simulink model "lab7_1"  (R2018b)
settings: Solver=VariableStepAuto  StartTime=0.0  StopTime=10.0  RelTol=1e-3
libraries: hdlsllib x86
(part 2 of 2)

== system lab7_1/Subsystem1/Full Adder2/Half Adder 1 ==
  note: Subsystem
  X : Inport
  Y : Inport  Port=2
  Logical Operator : Logic  IconShape=distinctive  AllPortsSameDT=off  OutDataTypeStr=boolean
  Logical Operator1 : Logic  Operator=XOR  IconShape=distinctive  AllPortsSameDT=off  OutDataTypeStr=boolean
  S : Outport
  C : Outport  Port=2
  wires:
  X/1 -> Logical Operator/1, Logical Operator1/1
  Y/1 -> Logical Operator1/2, Logical Operator/2
  Logical Operator/1 -> C/1
  Logical Operator1/1 -> S/1

== system lab7_1/Subsystem1/Full Adder3/Half Adder ==
  note: Subsystem
  X : Inport
  Y : Inport  Port=2
  Logical Operator : Logic  IconShape=distinctive  AllPortsSameDT=off  OutDataTypeStr=boolean
  Logical Operator1 : Logic  Operator=XOR  IconShape=distinctive  AllPortsSameDT=off  OutDataTypeStr=boolean
  S : Outport
  C : Outport  Port=2
  wires:
  X/1 -> Logical Operator/1, Logical Operator1/1
  Y/1 -> Logical Operator1/2, Logical Operator/2
  Logical Operator/1 -> C/1
  Logical Operator1/1 -> S/1

== system lab7_1/Subsystem1/Full Adder3/Half Adder 1 ==
  note: Subsystem
  X : Inport
  Y : Inport  Port=2
  Logical Operator : Logic  IconShape=distinctive  AllPortsSameDT=off  OutDataTypeStr=boolean
  Logical Operator1 : Logic  Operator=XOR  IconShape=distinctive  AllPortsSameDT=off  OutDataTypeStr=boolean
  S : Outport
  C : Outport  Port=2
  wires:
  X/1 -> Logical Operator/1, Logical Operator1/1
  Y/1 -> Logical Operator1/2, Logical Operator/2
  Logical Operator/1 -> C/1
  Logical Operator1/1 -> S/1

== system lab7_1/Subsystem1/Full Adder4/Half Adder ==
  note: Subsystem
  X : Inport
  Y : Inport  Port=2
  Logical Operator : Logic  IconShape=distinctive  AllPortsSameDT=off  OutDataTypeStr=boolean
  Logical Operator1 : Logic  Operator=XOR  IconShape=distinctive  AllPortsSameDT=off  OutDataTypeStr=boolean
  S : Outport
  C : Outport  Port=2
  wires:
  X/1 -> Logical Operator/1, Logical Operator1/1
  Y/1 -> Logical Operator1/2, Logical Operator/2
  Logical Operator/1 -> C/1
  Logical Operator1/1 -> S/1

== system lab7_1/Subsystem1/Full Adder4/Half Adder 1 ==
  note: Subsystem
  X : Inport
  Y : Inport  Port=2
  Logical Operator : Logic  IconShape=distinctive  AllPortsSameDT=off  OutDataTypeStr=boolean
  Logical Operator1 : Logic  Operator=XOR  IconShape=distinctive  AllPortsSameDT=off  OutDataTypeStr=boolean
  S : Outport
  C : Outport  Port=2
  wires:
  X/1 -> Logical Operator/1, Logical Operator1/1
  Y/1 -> Logical Operator1/2, Logical Operator/2
  Logical Operator/1 -> C/1
  Logical Operator1/1 -> S/1

== system lab7_1/Subsystem1/Full Adder5/Half Adder ==
  note: Subsystem
  X : Inport
  Y : Inport  Port=2
  Logical Operator : Logic  IconShape=distinctive  AllPortsSameDT=off  OutDataTypeStr=boolean
  Logical Operator1 : Logic  Operator=XOR  IconShape=distinctive  AllPortsSameDT=off  OutDataTypeStr=boolean
  S : Outport
  C : Outport  Port=2
  wires:
  X/1 -> Logical Operator/1, Logical Operator1/1
  Y/1 -> Logical Operator1/2, Logical Operator/2
  Logical Operator/1 -> C/1
  Logical Operator1/1 -> S/1

== system lab7_1/Subsystem1/Full Adder5/Half Adder 1 ==
  note: Subsystem
  X : Inport
  Y : Inport  Port=2
  Logical Operator : Logic  IconShape=distinctive  AllPortsSameDT=off  OutDataTypeStr=boolean
  Logical Operator1 : Logic  Operator=XOR  IconShape=distinctive  AllPortsSameDT=off  OutDataTypeStr=boolean
  S : Outport
  C : Outport  Port=2
  wires:
  X/1 -> Logical Operator/1, Logical Operator1/1
  Y/1 -> Logical Operator1/2, Logical Operator/2
  Logical Operator/1 -> C/1
  Logical Operator1/1 -> S/1

== system lab7_1/Subsystem1/Full Adder6/Half Adder ==
  note: Subsystem
  X : Inport
  Y : Inport  Port=2
  Logical Operator : Logic  IconShape=distinctive  AllPortsSameDT=off  OutDataTypeStr=boolean
  Logical Operator1 : Logic  Operator=XOR  IconShape=distinctive  AllPortsSameDT=off  OutDataTypeStr=boolean
  S : Outport
  C : Outport  Port=2
  wires:
  X/1 -> Logical Operator/1, Logical Operator1/1
  Y/1 -> Logical Operator1/2, Logical Operator/2
  Logical Operator/1 -> C/1
  Logical Operator1/1 -> S/1

== system lab7_1/Subsystem1/Full Adder6/Half Adder 1 ==
  note: Subsystem
  X : Inport
  Y : Inport  Port=2
  Logical Operator : Logic  IconShape=distinctive  AllPortsSameDT=off  OutDataTypeStr=boolean
  Logical Operator1 : Logic  Operator=XOR  IconShape=distinctive  AllPortsSameDT=off  OutDataTypeStr=boolean
  S : Outport
  C : Outport  Port=2
  wires:
  X/1 -> Logical Operator/1, Logical Operator1/1
  Y/1 -> Logical Operator1/2, Logical Operator/2
  Logical Operator/1 -> C/1
  Logical Operator1/1 -> S/1

== system lab7_1/Subsystem1/Full Adder7/Half Adder ==
  note: Subsystem
  X : Inport
  Y : Inport  Port=2
  Logical Operator : Logic  IconShape=distinctive  AllPortsSameDT=off  OutDataTypeStr=boolean
  Logical Operator1 : Logic  Operator=XOR  IconShape=distinctive  AllPortsSameDT=off  OutDataTypeStr=boolean
  S : Outport
  C : Outport  Port=2
  wires:
  X/1 -> Logical Operator/1, Logical Operator1/1
  Y/1 -> Logical Operator1/2, Logical Operator/2
  Logical Operator/1 -> C/1
  Logical Operator1/1 -> S/1

== system lab7_1/Subsystem1/Full Adder7/Half Adder 1 ==
  note: Subsystem
  X : Inport
  Y : Inport  Port=2
  Logical Operator : Logic  IconShape=distinctive  AllPortsSameDT=off  OutDataTypeStr=boolean
  Logical Operator1 : Logic  Operator=XOR  IconShape=distinctive  AllPortsSameDT=off  OutDataTypeStr=boolean
  S : Outport
  C : Outport  Port=2
  wires:
  X/1 -> Logical Operator/1, Logical Operator1/1
  Y/1 -> Logical Operator1/2, Logical Operator/2
  Logical Operator/1 -> C/1
  Logical Operator1/1 -> S/1

== system lab7_1/Subsystem2/Full Adder/Half Adder ==
  note: Subsystem
  X : Inport
  Y : Inport  Port=2
  Logical Operator : Logic  IconShape=distinctive  AllPortsSameDT=off  OutDataTypeStr=boolean
  Logical Operator1 : Logic  Operator=XOR  IconShape=distinctive  AllPortsSameDT=off  OutDataTypeStr=boolean
  S : Outport
  C : Outport  Port=2
  wires:
  X/1 -> Logical Operator/1, Logical Operator1/1
  Y/1 -> Logical Operator1/2, Logical Operator/2
  Logical Operator/1 -> C/1
  Logical Operator1/1 -> S/1

== system lab7_1/Subsystem2/Full Adder/Half Adder 1 ==
  note: Subsystem
  X : Inport
  Y : Inport  Port=2
  Logical Operator : Logic  IconShape=distinctive  AllPortsSameDT=off  OutDataTypeStr=boolean
  Logical Operator1 : Logic  Operator=XOR  IconShape=distinctive  AllPortsSameDT=off  OutDataTypeStr=boolean
  S : Outport
  C : Outport  Port=2
  wires:
  X/1 -> Logical Operator/1, Logical Operator1/1
  Y/1 -> Logical Operator1/2, Logical Operator/2
  Logical Operator/1 -> C/1
  Logical Operator1/1 -> S/1

== system lab7_1/Subsystem2/Full Adder1/Half Adder ==
  note: Subsystem
  X : Inport
  Y : Inport  Port=2
  Logical Operator : Logic  IconShape=distinctive  AllPortsSameDT=off  OutDataTypeStr=boolean
  Logical Operator1 : Logic  Operator=XOR  IconShape=distinctive  AllPortsSameDT=off  OutDataTypeStr=boolean
  S : Outport
  C : Outport  Port=2
  wires:
  X/1 -> Logical Operator/1, Logical Operator1/1
  Y/1 -> Logical Operator1/2, Logical Operator/2
  Logical Operator/1 -> C/1
  Logical Operator1/1 -> S/1

== system lab7_1/Subsystem2/Full Adder1/Half Adder 1 ==
  note: Subsystem
  X : Inport
  Y : Inport  Port=2
  Logical Operator : Logic  IconShape=distinctive  AllPortsSameDT=off  OutDataTypeStr=boolean
  Logical Operator1 : Logic  Operator=XOR  IconShape=distinctive  AllPortsSameDT=off  OutDataTypeStr=boolean
  S : Outport
  C : Outport  Port=2
  wires:
  X/1 -> Logical Operator/1, Logical Operator1/1
  Y/1 -> Logical Operator1/2, Logical Operator/2
  Logical Operator/1 -> C/1
  Logical Operator1/1 -> S/1

== system lab7_1/Subsystem2/Full Adder2/Half Adder ==
  note: Subsystem
  X : Inport
  Y : Inport  Port=2
  Logical Operator : Logic  IconShape=distinctive  AllPortsSameDT=off  OutDataTypeStr=boolean
  Logical Operator1 : Logic  Operator=XOR  IconShape=distinctive  AllPortsSameDT=off  OutDataTypeStr=boolean
  S : Outport
  C : Outport  Port=2
  wires:
  X/1 -> Logical Operator/1, Logical Operator1/1
  Y/1 -> Logical Operator1/2, Logical Operator/2
  Logical Operator/1 -> C/1
  Logical Operator1/1 -> S/1

== system lab7_1/Subsystem2/Full Adder2/Half Adder 1 ==
  note: Subsystem
  X : Inport
  Y : Inport  Port=2
  Logical Operator : Logic  IconShape=distinctive  AllPortsSameDT=off  OutDataTypeStr=boolean
  Logical Operator1 : Logic  Operator=XOR  IconShape=distinctive  AllPortsSameDT=off  OutDataTypeStr=boolean
  S : Outport
  C : Outport  Port=2
  wires:
  X/1 -> Logical Operator/1, Logical Operator1/1
  Y/1 -> Logical Operator1/2, Logical Operator/2
  Logical Operator/1 -> C/1
  Logical Operator1/1 -> S/1

== system lab7_1/Subsystem2/Full Adder3/Half Adder ==
  note: Subsystem
  X : Inport
  Y : Inport  Port=2
  Logical Operator : Logic  IconShape=distinctive  AllPortsSameDT=off  OutDataTypeStr=boolean
  Logical Operator1 : Logic  Operator=XOR  IconShape=distinctive  AllPortsSameDT=off  OutDataTypeStr=boolean
  S : Outport
  C : Outport  Port=2
  wires:
  X/1 -> Logical Operator/1, Logical Operator1/1
  Y/1 -> Logical Operator1/2, Logical Operator/2
  Logical Operator/1 -> C/1
  Logical Operator1/1 -> S/1

== system lab7_1/Subsystem2/Full Adder3/Half Adder 1 ==
  note: Subsystem
  X : Inport
  Y : Inport  Port=2
  Logical Operator : Logic  IconShape=distinctive  AllPortsSameDT=off  OutDataTypeStr=boolean
  Logical Operator1 : Logic  Operator=XOR  IconShape=distinctive  AllPortsSameDT=off  OutDataTypeStr=boolean
  S : Outport
  C : Outport  Port=2
  wires:
  X/1 -> Logical Operator/1, Logical Operator1/1
  Y/1 -> Logical Operator1/2, Logical Operator/2
  Logical Operator/1 -> C/1
  Logical Operator1/1 -> S/1

== system lab7_1/Subsystem2/Full Adder4/Half Adder ==
  note: Subsystem
  X : Inport
  Y : Inport  Port=2
  Logical Operator : Logic  IconShape=distinctive  AllPortsSameDT=off  OutDataTypeStr=boolean
  Logical Operator1 : Logic  Operator=XOR  IconShape=distinctive  AllPortsSameDT=off  OutDataTypeStr=boolean
  S : Outport
  C : Outport  Port=2
  wires:
  X/1 -> Logical Operator/1, Logical Operator1/1
  Y/1 -> Logical Operator1/2, Logical Operator/2
  Logical Operator/1 -> C/1
  Logical Operator1/1 -> S/1

== system lab7_1/Subsystem2/Full Adder4/Half Adder 1 ==
  note: Subsystem
  X : Inport
  Y : Inport  Port=2
  Logical Operator : Logic  IconShape=distinctive  AllPortsSameDT=off  OutDataTypeStr=boolean
  Logical Operator1 : Logic  Operator=XOR  IconShape=distinctive  AllPortsSameDT=off  OutDataTypeStr=boolean
  S : Outport
  C : Outport  Port=2
  wires:
  X/1 -> Logical Operator/1, Logical Operator1/1
  Y/1 -> Logical Operator1/2, Logical Operator/2
  Logical Operator/1 -> C/1
  Logical Operator1/1 -> S/1

== system lab7_1/Subsystem2/Full Adder5/Half Adder ==
  note: Subsystem
  X : Inport
  Y : Inport  Port=2
  Logical Operator : Logic  IconShape=distinctive  AllPortsSameDT=off  OutDataTypeStr=boolean
  Logical Operator1 : Logic  Operator=XOR  IconShape=distinctive  AllPortsSameDT=off  OutDataTypeStr=boolean
  S : Outport
  C : Outport  Port=2
  wires:
  X/1 -> Logical Operator/1, Logical Operator1/1
  Y/1 -> Logical Operator1/2, Logical Operator/2
  Logical Operator/1 -> C/1
  Logical Operator1/1 -> S/1

== system lab7_1/Subsystem2/Full Adder5/Half Adder 1 ==
  note: Subsystem
  X : Inport
  Y : Inport  Port=2
  Logical Operator : Logic  IconShape=distinctive  AllPortsSameDT=off  OutDataTypeStr=boolean
  Logical Operator1 : Logic  Operator=XOR  IconShape=distinctive  AllPortsSameDT=off  OutDataTypeStr=boolean
  S : Outport
  C : Outport  Port=2
  wires:
  X/1 -> Logical Operator/1, Logical Operator1/1
  Y/1 -> Logical Operator1/2, Logical Operator/2
  Logical Operator/1 -> C/1
  Logical Operator1/1 -> S/1

== system lab7_1/Subsystem2/Full Adder6/Half Adder ==
  note: Subsystem
  X : Inport
  Y : Inport  Port=2
  Logical Operator : Logic  IconShape=distinctive  AllPortsSameDT=off  OutDataTypeStr=boolean
  Logical Operator1 : Logic  Operator=XOR  IconShape=distinctive  AllPortsSameDT=off  OutDataTypeStr=boolean
  S : Outport
  C : Outport  Port=2
  wires:
  X/1 -> Logical Operator/1, Logical Operator1/1
  Y/1 -> Logical Operator1/2, Logical Operator/2
  Logical Operator/1 -> C/1
  Logical Operator1/1 -> S/1

== system lab7_1/Subsystem2/Full Adder6/Half Adder 1 ==
  note: Subsystem
  X : Inport
  Y : Inport  Port=2
  Logical Operator : Logic  IconShape=distinctive  AllPortsSameDT=off  OutDataTypeStr=boolean
  Logical Operator1 : Logic  Operator=XOR  IconShape=distinctive  AllPortsSameDT=off  OutDataTypeStr=boolean
  S : Outport
  C : Outport  Port=2
  wires:
  X/1 -> Logical Operator/1, Logical Operator1/1
  Y/1 -> Logical Operator1/2, Logical Operator/2
  Logical Operator/1 -> C/1
  Logical Operator1/1 -> S/1

== system lab7_1/Subsystem2/Full Adder7/Half Adder ==
  note: Subsystem
  X : Inport
  Y : Inport  Port=2
  Logical Operator : Logic  IconShape=distinctive  AllPortsSameDT=off  OutDataTypeStr=boolean
  Logical Operator1 : Logic  Operator=XOR  IconShape=distinctive  AllPortsSameDT=off  OutDataTypeStr=boolean
  S : Outport
  C : Outport  Port=2
  wires:
  X/1 -> Logical Operator/1, Logical Operator1/1
  Y/1 -> Logical Operator1/2, Logical Operator/2
  Logical Operator/1 -> C/1
  Logical Operator1/1 -> S/1

== system lab7_1/Subsystem2/Full Adder7/Half Adder 1 ==
  note: Subsystem
  X : Inport
  Y : Inport  Port=2
  Logical Operator : Logic  IconShape=distinctive  AllPortsSameDT=off  OutDataTypeStr=boolean
  Logical Operator1 : Logic  Operator=XOR  IconShape=distinctive  AllPortsSameDT=off  OutDataTypeStr=boolean
  S : Outport
  C : Outport  Port=2
  wires:
  X/1 -> Logical Operator/1, Logical Operator1/1
  Y/1 -> Logical Operator1/2, Logical Operator/2
  Logical Operator/1 -> C/1
  Logical Operator1/1 -> S/1

== system lab7_1/Subsystem3/Full Adder/Half Adder ==
  note: Subsystem
  X : Inport
  Y : Inport  Port=2
  Logical Operator : Logic  IconShape=distinctive  AllPortsSameDT=off  OutDataTypeStr=boolean
  Logical Operator1 : Logic  Operator=XOR  IconShape=distinctive  AllPortsSameDT=off  OutDataTypeStr=boolean
  S : Outport
  C : Outport  Port=2
  wires:
  X/1 -> Logical Operator/1, Logical Operator1/1
  Y/1 -> Logical Operator1/2, Logical Operator/2
  Logical Operator/1 -> C/1
  Logical Operator1/1 -> S/1

== system lab7_1/Subsystem3/Full Adder/Half Adder 1 ==
  note: Subsystem
  X : Inport
  Y : Inport  Port=2
  Logical Operator : Logic  IconShape=distinctive  AllPortsSameDT=off  OutDataTypeStr=boolean
  Logical Operator1 : Logic  Operator=XOR  IconShape=distinctive  AllPortsSameDT=off  OutDataTypeStr=boolean
  S : Outport
  C : Outport  Port=2
  wires:
  X/1 -> Logical Operator/1, Logical Operator1/1
  Y/1 -> Logical Operator1/2, Logical Operator/2
  Logical Operator/1 -> C/1
  Logical Operator1/1 -> S/1

== system lab7_1/Subsystem3/Full Adder1/Half Adder ==
  note: Subsystem
  X : Inport
  Y : Inport  Port=2
  Logical Operator : Logic  IconShape=distinctive  AllPortsSameDT=off  OutDataTypeStr=boolean
  Logical Operator1 : Logic  Operator=XOR  IconShape=distinctive  AllPortsSameDT=off  OutDataTypeStr=boolean
  S : Outport
  C : Outport  Port=2
  wires:
  X/1 -> Logical Operator/1, Logical Operator1/1
  Y/1 -> Logical Operator1/2, Logical Operator/2
  Logical Operator/1 -> C/1
  Logical Operator1/1 -> S/1

== system lab7_1/Subsystem3/Full Adder1/Half Adder 1 ==
  note: Subsystem
  X : Inport
  Y : Inport  Port=2
  Logical Operator : Logic  IconShape=distinctive  AllPortsSameDT=off  OutDataTypeStr=boolean
  Logical Operator1 : Logic  Operator=XOR  IconShape=distinctive  AllPortsSameDT=off  OutDataTypeStr=boolean
  S : Outport
  C : Outport  Port=2
  wires:
  X/1 -> Logical Operator/1, Logical Operator1/1
  Y/1 -> Logical Operator1/2, Logical Operator/2
  Logical Operator/1 -> C/1
  Logical Operator1/1 -> S/1

== system lab7_1/Subsystem3/Full Adder2/Half Adder ==
  note: Subsystem
  X : Inport
  Y : Inport  Port=2
  Logical Operator : Logic  IconShape=distinctive  AllPortsSameDT=off  OutDataTypeStr=boolean
  Logical Operator1 : Logic  Operator=XOR  IconShape=distinctive  AllPortsSameDT=off  OutDataTypeStr=boolean
  S : Outport
  C : Outport  Port=2
  wires:
  X/1 -> Logical Operator/1, Logical Operator1/1
  Y/1 -> Logical Operator1/2, Logical Operator/2
  Logical Operator/1 -> C/1
  Logical Operator1/1 -> S/1

== system lab7_1/Subsystem3/Full Adder2/Half Adder 1 ==
  note: Subsystem
  X : Inport
  Y : Inport  Port=2
  Logical Operator : Logic  IconShape=distinctive  AllPortsSameDT=off  OutDataTypeStr=boolean
  Logical Operator1 : Logic  Operator=XOR  IconShape=distinctive  AllPortsSameDT=off  OutDataTypeStr=boolean
  S : Outport
  C : Outport  Port=2
  wires:
  X/1 -> Logical Operator/1, Logical Operator1/1
  Y/1 -> Logical Operator1/2, Logical Operator/2
  Logical Operator/1 -> C/1
  Logical Operator1/1 -> S/1

== system lab7_1/Subsystem3/Full Adder3/Half Adder ==
  note: Subsystem
  X : Inport
  Y : Inport  Port=2
  Logical Operator : Logic  IconShape=distinctive  AllPortsSameDT=off  OutDataTypeStr=boolean
  Logical Operator1 : Logic  Operator=XOR  IconShape=distinctive  AllPortsSameDT=off  OutDataTypeStr=boolean
  S : Outport
  C : Outport  Port=2
  wires:
  X/1 -> Logical Operator/1, Logical Operator1/1
  Y/1 -> Logical Operator1/2, Logical Operator/2
  Logical Operator/1 -> C/1
  Logical Operator1/1 -> S/1

== system lab7_1/Subsystem3/Full Adder3/Half Adder 1 ==
  note: Subsystem
  X : Inport
  Y : Inport  Port=2
  Logical Operator : Logic  IconShape=distinctive  AllPortsSameDT=off  OutDataTypeStr=boolean
  Logical Operator1 : Logic  Operator=XOR  IconShape=distinctive  AllPortsSameDT=off  OutDataTypeStr=boolean
  S : Outport
  C : Outport  Port=2
  wires:
  X/1 -> Logical Operator/1, Logical Operator1/1
  Y/1 -> Logical Operator1/2, Logical Operator/2
  Logical Operator/1 -> C/1
  Logical Operator1/1 -> S/1

== system lab7_1/Subsystem3/Full Adder4/Half Adder ==
  note: Subsystem
  X : Inport
  Y : Inport  Port=2
  Logical Operator : Logic  IconShape=distinctive  AllPortsSameDT=off  OutDataTypeStr=boolean
  Logical Operator1 : Logic  Operator=XOR  IconShape=distinctive  AllPortsSameDT=off  OutDataTypeStr=boolean
  S : Outport
  C : Outport  Port=2
  wires:
  X/1 -> Logical Operator/1, Logical Operator1/1
  Y/1 -> Logical Operator1/2, Logical Operator/2
  Logical Operator/1 -> C/1
  Logical Operator1/1 -> S/1

== system lab7_1/Subsystem3/Full Adder4/Half Adder 1 ==
  note: Subsystem
  X : Inport
  Y : Inport  Port=2
  Logical Operator : Logic  IconShape=distinctive  AllPortsSameDT=off  OutDataTypeStr=boolean
  Logical Operator1 : Logic  Operator=XOR  IconShape=distinctive  AllPortsSameDT=off  OutDataTypeStr=boolean
  S : Outport
  C : Outport  Port=2
  wires:
  X/1 -> Logical Operator/1, Logical Operator1/1
  Y/1 -> Logical Operator1/2, Logical Operator/2
  Logical Operator/1 -> C/1
  Logical Operator1/1 -> S/1

== system lab7_1/Subsystem3/Full Adder5/Half Adder ==
  note: Subsystem
  X : Inport
  Y : Inport  Port=2
  Logical Operator : Logic  IconShape=distinctive  AllPortsSameDT=off  OutDataTypeStr=boolean
  Logical Operator1 : Logic  Operator=XOR  IconShape=distinctive  AllPortsSameDT=off  OutDataTypeStr=boolean
  S : Outport
  C : Outport  Port=2
  wires:
  X/1 -> Logical Operator/1, Logical Operator1/1
  Y/1 -> Logical Operator1/2, Logical Operator/2
  Logical Operator/1 -> C/1
  Logical Operator1/1 -> S/1

== system lab7_1/Subsystem3/Full Adder5/Half Adder 1 ==
  note: Subsystem
  X : Inport
  Y : Inport  Port=2
  Logical Operator : Logic  IconShape=distinctive  AllPortsSameDT=off  OutDataTypeStr=boolean
  Logical Operator1 : Logic  Operator=XOR  IconShape=distinctive  AllPortsSameDT=off  OutDataTypeStr=boolean
  S : Outport
  C : Outport  Port=2
  wires:
  X/1 -> Logical Operator/1, Logical Operator1/1
  Y/1 -> Logical Operator1/2, Logical Operator/2
  Logical Operator/1 -> C/1
  Logical Operator1/1 -> S/1

== system lab7_1/Subsystem3/Full Adder6/Half Adder ==
  note: Subsystem
  X : Inport
  Y : Inport  Port=2
  Logical Operator : Logic  IconShape=distinctive  AllPortsSameDT=off  OutDataTypeStr=boolean
  Logical Operator1 : Logic  Operator=XOR  IconShape=distinctive  AllPortsSameDT=off  OutDataTypeStr=boolean
  S : Outport
  C : Outport  Port=2
  wires:
  X/1 -> Logical Operator/1, Logical Operator1/1
  Y/1 -> Logical Operator1/2, Logical Operator/2
  Logical Operator/1 -> C/1
  Logical Operator1/1 -> S/1

== system lab7_1/Subsystem3/Full Adder6/Half Adder 1 ==
  note: Subsystem
  X : Inport
  Y : Inport  Port=2
  Logical Operator : Logic  IconShape=distinctive  AllPortsSameDT=off  OutDataTypeStr=boolean
  Logical Operator1 : Logic  Operator=XOR  IconShape=distinctive  AllPortsSameDT=off  OutDataTypeStr=boolean
  S : Outport
  C : Outport  Port=2
  wires:
  X/1 -> Logical Operator/1, Logical Operator1/1
  Y/1 -> Logical Operator1/2, Logical Operator/2
  Logical Operator/1 -> C/1
  Logical Operator1/1 -> S/1

== system lab7_1/Subsystem3/Full Adder7/Half Adder ==
  note: Subsystem
  X : Inport
  Y : Inport  Port=2
  Logical Operator : Logic  IconShape=distinctive  AllPortsSameDT=off  OutDataTypeStr=boolean
  Logical Operator1 : Logic  Operator=XOR  IconShape=distinctive  AllPortsSameDT=off  OutDataTypeStr=boolean
  S : Outport
  C : Outport  Port=2
  wires:
  X/1 -> Logical Operator/1, Logical Operator1/1
  Y/1 -> Logical Operator1/2, Logical Operator/2
  Logical Operator/1 -> C/1
  Logical Operator1/1 -> S/1

== system lab7_1/Subsystem3/Full Adder7/Half Adder 1 ==
  note: Subsystem
  X : Inport
  Y : Inport  Port=2
  Logical Operator : Logic  IconShape=distinctive  AllPortsSameDT=off  OutDataTypeStr=boolean
  Logical Operator1 : Logic  Operator=XOR  IconShape=distinctive  AllPortsSameDT=off  OutDataTypeStr=boolean
  S : Outport
  C : Outport  Port=2
  wires:
  X/1 -> Logical Operator/1, Logical Operator1/1
  Y/1 -> Logical Operator1/2, Logical Operator/2
  Logical Operator/1 -> C/1
  Logical Operator1/1 -> S/1
